simulink model "Simple_lin_model"  (R2023a)
settings: Solver=VariableStepAuto  StartTime=0.0  StopTime=4  FixedStep=0.01  MaxStep=0.01  RelTol=1e-4
undefined symbols (not defined in the file): i, J_rot, Jk, K_m, K_omega, R_3ph, T_q
settings Model: Creator=Artem Sannikov  LastModifiedBy=Artem Sannikov

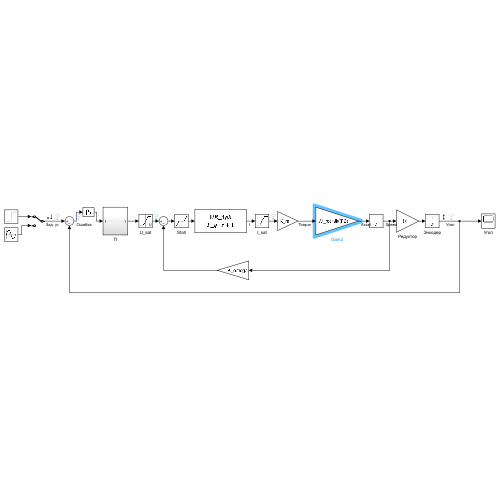
[thumbnail: Simulink's stored preview of the top-level diagram]
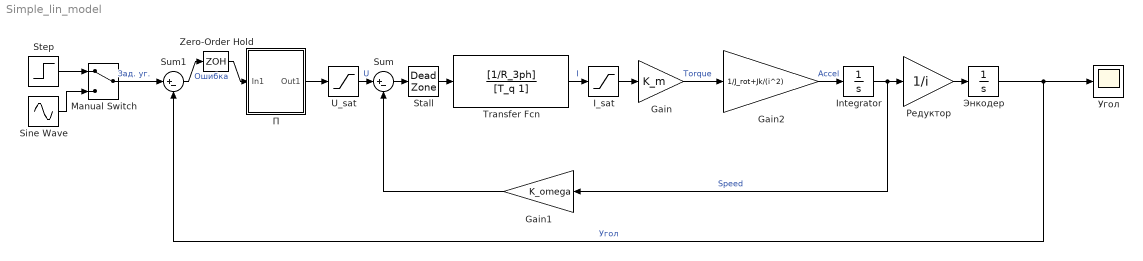
== system Simple_lin_model ==
  Gain : Gain  Gain=K_m
  Gain1 : Gain  Gain=K_omega
  Gain2 : Gain  Gain=1/J_rot+Jk/(i^2)
  I_sat : Saturate  UpperLimit=4  LowerLimit=-4
  Integrator : Integrator
  Manual Switch : ManualSwitch
  Sine Wave : Sin  Amplitude=8.72  Frequency=10  SampleTime=0
  Stall : DeadZone  LowerValue=-5  UpperValue=5
  Step : Step  SampleTime=0
  Sum : Sum  Inputs=|+-
  Sum1 : Sum  Inputs=|+-
  Transfer Fcn : TransferFcn  Numerator=[1/R_3ph]  Denominator=[T_q 1]
  U_sat : Saturate  UpperLimit=11.8  LowerLimit=-11.8
  Zero-Order Hold : ZeroOrderHold  SampleTime=0.001
  П : Subsystem
  Редуктор : Gain  Gain=1/i
  Угол : Scope
  Энкодер : Integrator
  wires:
  Gain1/1 -> Sum/2
  Transfer Fcn/1 -> I_sat/1  "I"
  Gain/1 -> Gain2/1  "Torque"
  Gain2/1 -> Integrator/1  "Accel"
  Integrator/1 -> Gain1/1, Редуктор/1  "Speed"
  Редуктор/1 -> Энкодер/1
  Энкодер/1 -> Sum1/2, Угол/1  "Угол"
  Step/1 -> Manual Switch/1
  Sine Wave/1 -> Manual Switch/2
  Manual Switch/1 -> Sum1/1  "Зад. уг."
  I_sat/1 -> Gain/1
  U_sat/1 -> Sum/1  "U"
  Sum/1 -> Stall/1
  Stall/1 -> Transfer Fcn/1
  П/1(Out1) -> U_sat/1
  Sum1/1 -> Zero-Order Hold/1  "Ошибка"
  Zero-Order Hold/1 -> П/1(In1)

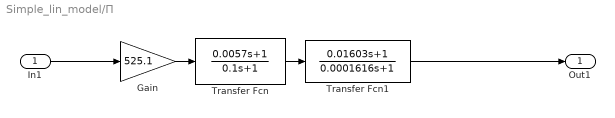
== system Simple_lin_model/П ==
  In1 : Inport
  Gain : Gain  Gain=525.1
  Transfer Fcn : TransferFcn  Numerator=[0.0057 1]  Denominator=[0.1 1]
  Transfer Fcn1 : TransferFcn  Numerator=[0.01603 1]  Denominator=[0.0001616 1]
  Out1 : Outport
  wires:
  Gain/1 -> Transfer Fcn/1
  Transfer Fcn/1 -> Transfer Fcn1/1
  In1/1 -> Gain/1
  Transfer Fcn1/1 -> Out1/1
